simulink model "sedemo_pulse_width_mod"  (Simulink 7.5)
settings: Solver=VariableStepDiscrete  StartTime=0.0  StopTime=1e-8  MaxStep=inf  RelTol=1e-3
libraries: simulink x2, simeventstranslate1 x2, simeventsinfo x1
settings Model: Creator=The MathWorks Inc.  ExtModeAutoUpdateStatusClock=off
settings DataIOCC: SaveOutput=off  SignalLogging=off  SaveTime=off
settings OptimizationCC: InitFltsAndDblsToZero=on
settings DebuggingCC: AlgebraicLoopMsg=error  SignalResolutionControl=TryResolveAllWithWarning  SolverPrmCheckMsg=none  StrictBusMsg=Warning
settings GRTTargetCC: TargetFcnLib=ansi_tfl_tmw_new.mat
settings SimEventsCC: propDiagAttribOutput=1  propDiagFcnCallOutput=1  propDiagStatOutput=0

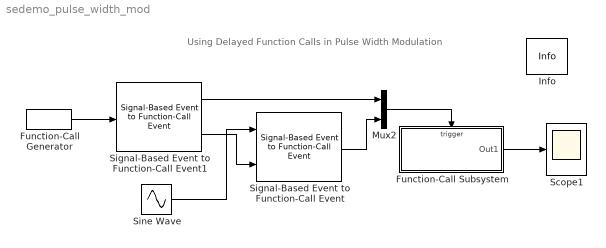
== system sedemo_pulse_width_mod ==
  note: Using Delayed Function Calls
      |  in Pulse Width Modulation
  Function-Call Generator : simulink/Ports & Subsystems/Function-Call Generator  sample_time=1e-10  numberOfIterations=1
  Function-Call Subsystem : Subsystem  TreatAsAtomicUnit=on
      settings: PropExecContextOutsideSubsystem=on
  Info : simeventsinfo/Info  SystemSampleTime=-1
  Mux2 : Mux  Inputs=2
  Scope1 : Scope
      settings: TimeRange=1e-08  YMin=-0.2  YMax=1.2
  Signal-Based Event to Function-Call Event : simeventstranslate1/Signal-Based Event to Function-Call Event  Priority=1  SystemSampleTime=-1  GenerateFunctionCallUpon=Function call from port fcn  SignalEdgeOption=Rising  EnableE1Port=off  EnableF2Port=off  EnableE2Port=off  SpecifyEventPriority=on  PriorityFunctionCall=200  FunctionCallDelayFrom=Signal port t  DelayFunctionCall=0  StatNumberF1Calls=Off  StatNumberF2Calls=Off  MaskBlockType=none
  Signal-Based Event to Function-Call Event1 : simeventstranslate1/Signal-Based Event to Function-Call Event  Priority=1  SystemSampleTime=-1  GenerateFunctionCallUpon=Function call from port fcn  SignalEdgeOption=Rising  EnableE1Port=off  EnableF2Port=on  EnableE2Port=off  SpecifyEventPriority=off  PriorityFunctionCall=200  FunctionCallDelayFrom=Signal port t  DelayFunctionCall=0  StatNumberF1Calls=Off  StatNumberF2Calls=Off  MaskBlockType=none
  Sine Wave : Sin  Amplitude=1e-10  Bias=1e-10 + eps  Frequency=2*pi*1e8  Phase=0  Samples=10  SampleTime=0  Offset=0
  wires:
  Function-Call Generator/1 -> Signal-Based Event to Function-Call Event1/1
  Signal-Based Event to Function-Call Event1/2 -> Signal-Based Event to Function-Call Event/2
  Signal-Based Event to Function-Call Event1/1 -> Mux2/1
  Signal-Based Event to Function-Call Event/1 -> Mux2/2
  Mux2/1 -> Function-Call Subsystem/Trigger
  Sine Wave/1 -> Signal-Based Event to Function-Call Event/1
  Function-Call Subsystem/1(Out1) -> Scope1/1

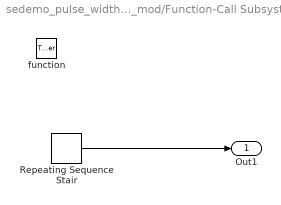
== system sedemo_pulse_width_mod/Function-Call Subsystem ==
  function : TriggerPort  TriggerType=function-call
  Repeating Sequence Stair : simulink/Sources/Repeating Sequence Stair  SystemSampleTime=-1  OutValues=[1 0].'  tsamp=-1  OutputDataTypeScalingMode=Specify via dialog  OutDataType=float('double')  ConRadixGroup=Best Precision: Vector-wise  OutScaling=2^-12
  Out1 : Outport  OutDataType=sfix(16)  OutScaling=2^0
  wires:
  Repeating Sequence Stair/1 -> Out1/1
